simulink model "pando_MPPT"  (R2020a)
settings: Solver=VariableStepAuto  StartTime=0.0  StopTime=10.0  RelTol=1e-3
undefined symbols (not defined in the file): sigbuilder_block, StepSize
libraries: powerlib x12, re_lib x1, powerlib_meascontrol x1
settings Model: Creator=sameeraa  LastModifiedBy=sameeraa

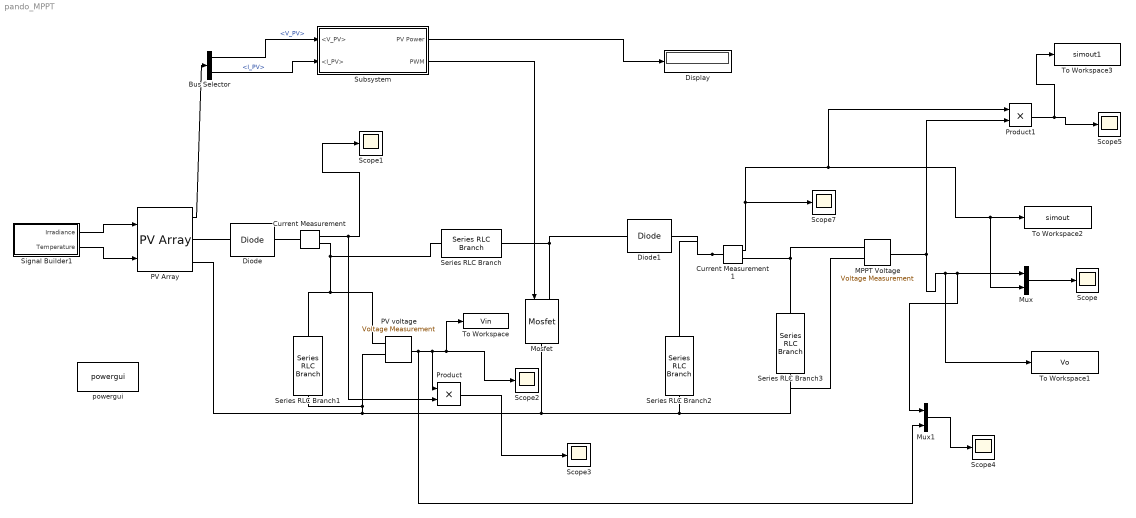
== system pando_MPPT ==
  Bus Selector : BusSelector  OutputSignals=V_PV,I_PV
  Current Measurement : powerlib/Measurements/Current Measurement  PhasorSimulation=off  OutputType=Complex  PSBequivalent=0
  Current Measurement1 : powerlib/Measurements/Current Measurement  PhasorSimulation=off  OutputType=Complex  PSBequivalent=0
  Diode : powerlib/Power Electronics/Diode  Ron=0.001  Lon=0  Vf=0.8  IC=0  UseSnubber=0  Rs=500  Cs=250e-9  Measurements=off
  Diode1 : powerlib/Power Electronics/Diode  Ron=0.001  Lon=0  Vf=0.8  IC=0  UseSnubber=0  Rs=500  Cs=250e-9  Measurements=off
  Display : Display
  MPPT Voltage : powerlib/Measurements/Voltage Measurement  PhasorSimulation=off  OutputType=Complex  PSBequivalent=0
  Mosfet : powerlib/Power Electronics/Mosfet  Ron=0.1  Lon=0  Rd=0.01  Vfd=0  IC=0  Rs=1e5  Cs=inf  Measurements=off
  Mux : Mux  Inputs=2
  Mux1 : Mux  Inputs=2
  PV Array : re_lib/Solar/PV Array  Npar=1  Nser=1  PlotType=one module @ 25 deg.C & specified irradiances  S_vec="[ 1000  800  600 ]"  Temp_C_vec="[ 45 25  ]"  ModuleName=User-defined  PlotWhenSelected=off  Pm=223.3  Ncell=60  Voc=36.3  Isc=7.84  Vm=29  Im=7.7  beta_Voc_pc=-0.36099  alpha_Isc_pc=0.102  beta_Voc=-0.13104  alpha_Isc=0.0079968  IL=8.0515  I0=2.9406e-10  nI=0.97985  Rsh=6175.6519  Rs=0.38059  RobustModel=off  RobustCellTemperature=25  BAL=on  Tc=1e-6  Tfilter=5e-5
  PV voltage : powerlib/Measurements/Voltage Measurement  PhasorSimulation=off  OutputType=Complex  PSBequivalent=0
  Product : Product
  Product1 : Product
  Scope{,1..5,7} (7 alike) : Scope
  Series RLC Branch : powerlib/Elements/Series RLC Branch  LConnTagsString=__new0  RConnTagsString=__new0  BranchType=L  Resistance=1  Inductance=1e-3  SetiL0=off  InitialCurrent=0  Capacitance=1e-6  Setx0=off  InitialVoltage=0  Measurements=None
  Series RLC Branch1 : powerlib/Elements/Series RLC Branch  LConnTagsString=__new0  RConnTagsString=__new0  BranchType=C  Resistance=1  Inductance=1e-3  SetiL0=off  InitialCurrent=0  Capacitance=1e-6  Setx0=off  InitialVoltage=0  Measurements=None
  Series RLC Branch2 : powerlib/Elements/Series RLC Branch  LConnTagsString=__new0  RConnTagsString=__new0  BranchType=C  Resistance=1  Inductance=1e-3  SetiL0=off  InitialCurrent=0  Capacitance=1e-6  Setx0=off  InitialVoltage=0  Measurements=None
  Series RLC Branch3 : powerlib/Elements/Series RLC Branch  LConnTagsString=__new0  RConnTagsString=__new0  BranchType=R  Resistance=1  Inductance=1e-3  SetiL0=off  InitialCurrent=0  Capacitance=1e-6  Setx0=off  InitialVoltage=0  Measurements=None
  Signal Builder1 : Subsystem  Tag=STV Subsys  LoadFcn=sigbuilder_block('load');  StartFcn=sigbuilder_block('start');  StopFcn=sigbuilder_block('stop');  ClipboardFcn=sigbuilder_block('clipboard');  mask(Sigbuilder block){tuvar=[0:10]}
      mask help: Simulink:masks:SigbuilderBlock_MD
      mask init:
      | if ~strcmp(get_param(bdroot(gcbh),'SimulationStatus'),'stopped') tuvar = sigbuilder_block('maskInit'); end
      settings: CopyFcn=sigbuilder_block('copy');  DeleteFcn=sigbuilder_block('delete');  ModelCloseFcn=sigbuilder_block('modelClose');  PreSaveFcn=sigbuilder_block('preSave');  PauseFcn=sigbuilder_block('pause');  ContinueFcn=sigbuilder_block('continue');  NameChangeFcn=sigbuilder_block('namechange');  OpenFcn=sigbuilder_block('open',[382.8 123 550.8 400.2 ]);  CloseFcn=sigbuilder_block('close');
      mask Display: plot(0, 0, 100, 100,[2, 2, 32, 32, 2], [68, 8, 8, 68, 68],[32, 2], [38, 38], [32, 19, 2],[53, 60, 44], [32, 17, 17, 2],[16, 16, 31, 31]);txt = getActiveGroup(gcbh);text(2, 100, txt,'verticalAlignment', 'top');
  Subsystem : Subsystem
  To Workspace : ToWorkspace  VariableName=Vin  SampleTime=-1
  To Workspace1 : ToWorkspace  VariableName=Vo  SampleTime=-1
  To Workspace2 : ToWorkspace  VariableName=simout  SaveFormat=Timeseries  SampleTime=-1
  To Workspace3 : ToWorkspace  VariableName=simout1  SaveFormat=Timeseries  SampleTime=-1
  powergui : powerlib/powergui  Priority=1  SimulationMode=Continuous  SampleTime=50e-6  frequency=60  Iterations=50  frequencyindice=0  Pbase=100e6  ErrMax=1e-4  UnitsV=kV  UnitsW=MW  buscounter=0  FunctionMessages=off  echomessages=off  EnableUseOfTLC=off  CurrentSourceSwitches=off  DisableSnubberDevices=off  DisableRonSwitches=off  DisableVfSwitches=off  DisplayEquations=off  AutomaticDiscreteSolvers=off  SolverType=Tustin/Backward Euler (TBE)  Interpol=off  ExternalGateDelay=off  methode=off  Ts=100  x0status=blocks  SPID=on  SwTol=0  HookPort=off  NonlinearTolerance=1e-4  nMaxIteration=100  ContinueOnMaxIteration=off  RestoreLinks=warning  ResistiveCurrentMeasurement=off  Frange=[0:2:500]  Ylog=off  Xlog=on  ShowGrid=off  save=off  variable=ZData  structure=0  ZoomFFT=off  StartTime=0.0  cycles=1  DisplayStyle=1  fundamental=60  FreqAxis=off  MaxFrequency=1000  frequencyindicesteady=1  RmsSteady=1  display=off
  wires:
  Product1/1 -> To Workspace3/1, Scope5/1
  Current Measurement1/1 -> Scope7/1, Product1/1, To Workspace2/1, Mux/2
  Product/1 -> Scope3/1
  Mux1/1 -> Scope4/1
  Current Measurement/1 -> Product/2, Scope1/1
  MPPT Voltage/1 -> To Workspace1/1, Mux/1, Mux1/1, Product1/2
  Signal Builder1/2(Temperature) -> PV Array/2
  Mux/1 -> Scope/1
  Signal Builder1/1(Irradiance) -> PV Array/1
  PV voltage/1 -> Scope2/1, To Workspace/1, Product/1, Mux1/2
  Subsystem/1(PV Power) -> Display/1
  PV Array/1 -> Bus Selector/1
  Subsystem/2(PWM) -> Mosfet/1
  Bus Selector/1 -> Subsystem/1(<V_PV>)  "<V_PV>"
  Bus Selector/2 -> Subsystem/2(<I_PV>)  "<I_PV>"
  connections:
  Series RLC Branch1/LConn1 -- PV voltage/LConn1 -- Series RLC Branch/LConn1 -- Current Measurement/RConn1
  Series RLC Branch2/RConn1 -- PV Array/RConn2 -- PV voltage/LConn2 -- Series RLC Branch1/RConn1 -- Mosfet/RConn1 -- MPPT Voltage/LConn2 -- Series RLC Branch3/RConn1
  Current Measurement1/LConn1 -- Diode1/RConn1 -- Series RLC Branch2/LConn1
  MPPT Voltage/LConn1 -- Current Measurement1/RConn1 -- Series RLC Branch3/LConn1
  Mosfet/LConn1 -- Series RLC Branch/RConn1 -- Diode1/LConn1
  Diode/RConn1 -- Current Measurement/LConn1
  PV Array/RConn1 -- Diode/LConn1

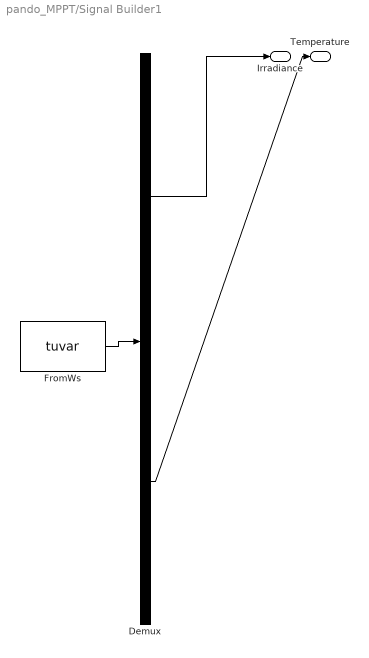
== system pando_MPPT/Signal Builder1 ==
  Demux : Demux  Tag=STV Demux  Outputs=2
      settings: DisplayOption=none
  FromWs : FromWorkspace  Tag=STV FromWs  VariableName=tuvar
      SigBuilderData=|
      | common.afterFinalStr = 'Extrapolate'
      | common.sampleTime = 0
      | dataSet.timeRange = [0 10]
      | dataSet.name = 'Group 1'
      | sbobj.Groups.Name = 'Group 1'
      | sbobj.Groups.Signals(1).Name = 'Irradiance'
      | sbobj.Groups.Signals(1).XData = [0 10]
      | sbobj.Groups.Signals(1).YData = [1000 1000]
      | sbobj.Groups.Signals(2).Name = 'Temperature'
      | sbobj.Groups.Signals(2).XData = [0 10]
      | sbobj.Groups.Signals(2).YData = [25 25]
  Irradiance : Outport  Tag=STV Outport
  Temperature : Outport  Tag=STV Outport  Port=2
  wires:
  Demux/1 -> Irradiance/1
  FromWs/1 -> Demux/1
  Demux/2 -> Temperature/1

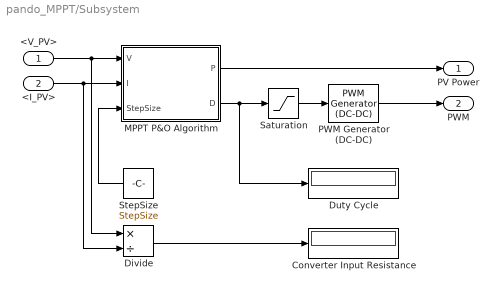
== system pando_MPPT/Subsystem ==
  <V_PV> : Inport
  <I_PV> : Inport  Port=2
  Converter Input Resistance : Display
  Divide : Product  Inputs=*/
  Duty Cycle : Display
  MPPT P&O Algorithm : MATLAB Function  TreatAsAtomicUnit=on
  PWM Generator (DC-DC) : powerlib_meascontrol/Pulse & Signal Generators/PWM Generator (DC-DC)  Fsw=Fsw  Ts=0
  Saturation : Saturate  UpperLimit=1  LowerLimit=0
  StepSize : Constant  Value=StepSize
  PV Power : Outport  VectorParamsAs1DForOutWhenUnconnected=off
  PWM : Outport  Port=2  VectorParamsAs1DForOutWhenUnconnected=off
  wires:
  Divide/1 -> Converter Input Resistance/1
  <I_PV>/1 -> MPPT P&O Algorithm/2(I), Divide/2
  MPPT P&O Algorithm/2(D) -> Saturation/1, Duty Cycle/1
  Saturation/1 -> PWM Generator (DC-DC)/1
  <V_PV>/1 -> MPPT P&O Algorithm/1(V), Divide/1
  PWM Generator (DC-DC)/1 -> PWM/1
  MPPT P&O Algorithm/1(P) -> PV Power/1
  StepSize/1 -> MPPT P&O Algorithm/3(StepSize)

== matlab function pando_MPPT/Subsystem/MPPT P&O Algorithm ==
  settings: updateMethod=DISCRETE
  data: P output; V input; D output; I input; StepSize input
function [P, D] = fcn(V,I,StepSize)
    % Initialization
    persistent Pprev Vprev Dprev
    if isempty(Pprev)
        Pprev = 0;
        Vprev = 0;
        Dprev = 0.5;
    end
    % P&O Algorithm Begin here
    P = I*V;
    if (P-Pprev) > 0
        if (V-Vprev) > 0
            D = Dprev - StepSize;
        else
            D = Dprev + StepSize;
        end
    else
        if (V-Vprev) > 0
            D = Dprev + StepSize;
        else
            D = Dprev - StepSize;
        end
    end
    % Update current value to previous value
    Pprev = P;
    Vprev = V;
    Dprev = D;
end
